simulink model "Lab5"  (R2018a)
settings: Solver=FixedStepDiscrete  StartTime=0.0  StopTime=10  FixedStep=1e-4  RelTol=1e-3
settings Model: Creator=cvillal3  LastModifiedBy=cvillal3

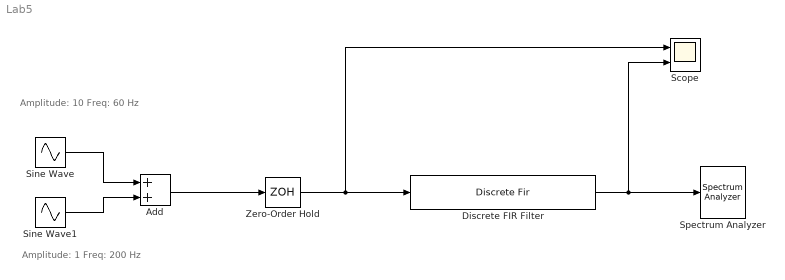
== system Lab5 ==
  note: Amplitude: 1
      | Freq: 200 Hz
  note: Amplitude: 10
      | Freq: 60 Hz
  Add : Sum
  Discrete FIR Filter : DiscreteFir  Coefficients=[0.325 -0.325*1.458 0.325]
  Scope : Scope  NumInputPorts=2
  Sine Wave : Sin  Amplitude=10  Frequency=60*2*pi  SampleTime=0
  Sine Wave1 : Sin  Frequency=200*2*pi  SampleTime=0
  Spectrum Analyzer : SpectrumAnalyzer
  Zero-Order Hold : ZeroOrderHold  SampleTime=1/500
  wires:
  Discrete FIR Filter/1 -> Scope/2, Spectrum Analyzer/1
  Sine Wave/1 -> Add/1
  Sine Wave1/1 -> Add/2
  Add/1 -> Zero-Order Hold/1
  Zero-Order Hold/1 -> Scope/1, Discrete FIR Filter/1
